simulink model "inverse_dynamics_2dof_PID"  (R2023b)
settings: Solver=VariableStepAuto  StartTime=0.0  StopTime=Tend_slk  RelTol=1e-3
values from neighbouring files (symbols this model uses):
  Kd11 = 0.01333    [main_inverse_2dof_PID.m]
  Kd22 = 0.01333    [main_inverse_2dof_PID.m]
  Ki11 = 7.259e-10    [main_inverse_2dof_PID.m]
  Ki22 = 7.259e-10    [main_inverse_2dof_PID.m]
  Kp11 = 6.221e-06    [main_inverse_2dof_PID.m]
  Kp22 = 6.221e-06    [main_inverse_2dof_PID.m]
  param = [Ixx;Iyy;Izz;l;k1;k2;k3;k4;b;m]    [main_inverse_2dof_PID.m]
  Ts_slk = 0.01    [main_inverse_2dof_PID.m]
  x0 = [0;0;0;0]    [main_inverse_2dof_PID.m]
undefined symbols (not defined in the file or in its folder): x_eq
libraries: slpidlib x2, cstblocks x1
settings Model: Creator=asus  LastModifiedBy=asus
settings OptimizationCC: ReuseModelBlockBuffer=off

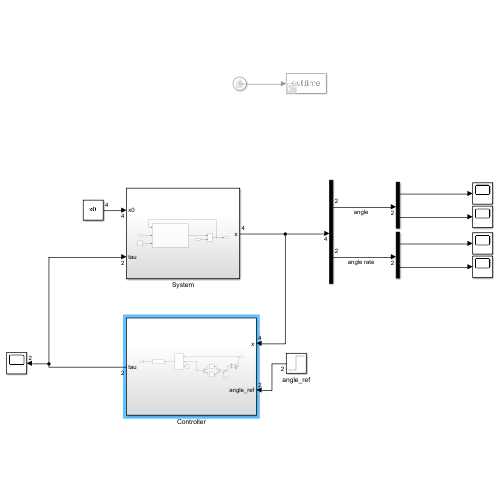
[thumbnail: Simulink's stored preview of the top-level diagram]
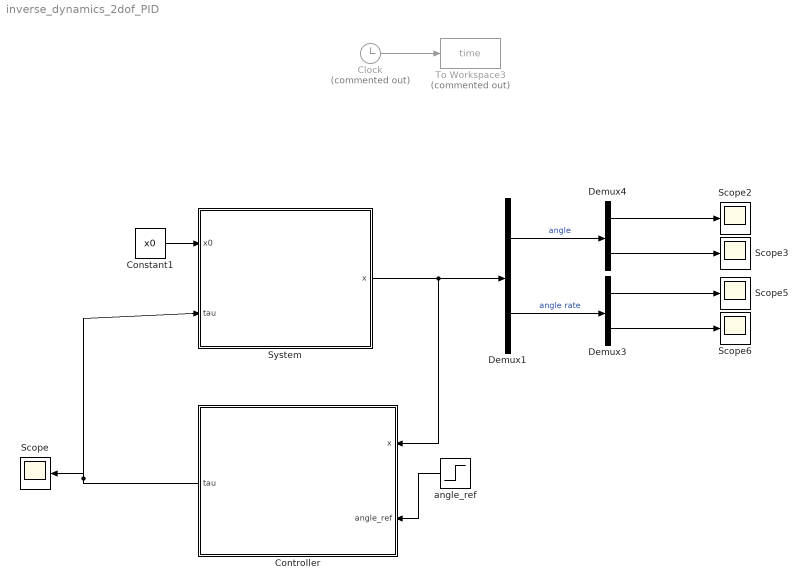
== system inverse_dynamics_2dof_PID ==
  Clock : Clock  Commented=on
  Constant1 : Constant  Value=x0
  Controller : Subsystem
  Demux1 : Demux  Outputs=2
  Demux3 : Demux  Outputs=2
  Demux4 : Demux  Outputs=2
  Scope{,2..3,5..6} (5 alike) : Scope
  System : Subsystem
  To Workspace3 : ToWorkspace  Commented=on  VariableName=time  SampleTime=Ts_slk
      settings: Save2DSignal=2-D array (concatenate along first dimension)
  angle_ref : Step  Time=0  After=[1;1]*30*pi/180  SampleTime=0
  wires:
  Clock/1 -> To Workspace3/1
  Demux4/1 -> Scope2/1
  Demux3/1 -> Scope5/1
  Demux4/2 -> Scope3/1
  Demux3/2 -> Scope6/1
  System/1(x) -> Controller/1(x), Demux1/1
  Demux1/2 -> Demux3/1  "angle rate"
  Demux1/1 -> Demux4/1  "angle"
  Controller/1(tau) -> Scope/1, System/2("tau ")
  angle_ref/1 -> Controller/2(angle_ref)
  Constant1/1 -> System/1(x0)

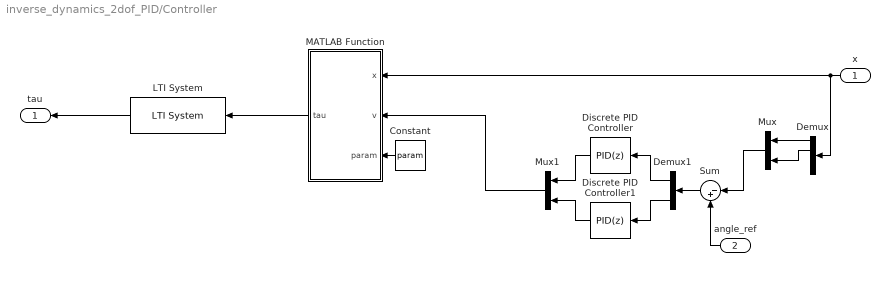
== system inverse_dynamics_2dof_PID/Controller ==
  x : Inport
  angle_ref : Inport  Port=2
  Constant : Constant  Value=param
  Demux : Demux
  Demux1 : Demux  Outputs=2
  Discrete PID Controller : slpidlib/PID Controller  Controller=PID  Form=Parallel  TimeDomain=Discrete-time  UseExternalTs=off  SampleTime=-1  IntegratorMethod=Forward Euler  FilterMethod=Forward Euler  ControllerParametersSource=internal  P=Kp11  I=Ki11  UseKiTs=off  D=Kd11  N=100  UseFilter=on  TunerSelectOption=Transfer Function Based (PID Tuner App)  InitialConditionSource=internal  InitialConditionForIntegrator=0  InitialConditionForFilter=0  DifferentiatorICPrevScaledInput=0  ExternalReset=none  TrackingMode=off  Kt=1  LimitOutput=off  SatLimitsSource=internal  UpperSaturationLimit=inf  LowerSaturationLimit=-inf  LinearizeAsGain=off  AntiWindupMode=none  Kb=1  LimitIntegrator=off  UpperIntegratorSaturationLimit=inf  LowerIntegratorSaturationLimit=-inf  POutMin=[]  POutMax=[]  IOutMin=[]  IOutMax=[]  DOutMin=[]  DOutMax=[]  NOutMin=[]  NOutMax=[]  SumOutMin=[]  SumOutMax=[]  SaturationOutMin=[]  SaturationOutMax=[]  PParamMin=[]  PParamMax=[]  IParamMin=[]  IParamMax=[]  DParamMin=[]  DParamMax=[]  NParamMin=[]  NParamMax=[]  KbParamMin=[]  KbParamMax=[]  KtParamMin=[]  KtParamMax=[]  KbOutMin=[]  KbOutMax=[]  KtOutMin=[]  KtOutMax=[]  IntegratorOutMin=[]  IntegratorOutMax=[]  FilterOutMin=[]  FilterOutMax=[]  SumI1OutMin=[]  SumI1OutMax=[]  SumI2OutMin=[]  SumI2OutMax=[]  SumI3OutMin=[]  SumI3OutMax=[]  SumI4OutMin=[]  SumI4OutMax=[]  SumDOutMin=[]  SumDOutMax=[]  DifferentiatorOutMin=[]  DifferentiatorOutMax=[]  FilterDiffOutCoefMin=[]  FilterDiffOutCoefMax=[]  ReciprocalOutMin=[]  ReciprocalOutMax=[]  SumDenOutMin=[]  SumDenOutMax=[]  SumNumOutMin=[]  SumNumOutMax=[]  DivideOutMin=[]  DivideOutMax=[]  UdiffTsProdOutMin=[]  UdiffTsProdOutMax=[]  NTsProdOutMin=[]  NTsProdOutMax=[]  UintegralTsProdOutMin=[]  UintegralTsProdOutMax=[]  UngainTsProdOutMin=[]  UngainTsProdOutMax=[]  ClampingZeroOutDataTypeStr=Inherit: Inherit via back propagation  ClampingZeroOutMin=[]  ClampingZeroOutMax=[]  FilterDenConstantOutDataTypeStr=Inherit: Inherit via back propagation  FilterDenConstantOutMin=[]  FilterDenConstantOutMax=[]  PCopyOutDataTypeStr=Inherit: Inherit via back propagation  PCopyOutMin=[]  PCopyOutMax=[]  NCopyOutDataTypeStr=Inherit: Inherit via back propagation  NCopyOutMin=[]  NCopyOutMax=[]  IntegratorContinuousStateAttributes=''  IntegratorStateMustResolveToSignalObject=off  IntegratorRTWStateStorageClass=Auto  FilterContinuousStateAttributes=''  FilterStateMustResolveToSignalObject=off  FilterRTWStateStorageClass=Auto  ParallelPVariant=InternalParameters  IdealPVariant=Disabled  IVariant=InternalParameters  DVariant=InternalParameters  IntegratorVariant=Discrete  SatVariant=Disabled  AWVariant=Passthrough  PCopyVariant=Disabled  TRVariant=Disabled  FdbkBlocksVariant=Forward  IdealPFdbkVariant=Disabled  SatFdbkVariant=Disabled  DerivativeFilterVariant=ForwardEulerFilter  NVariant=InternalParameters  NCopyVariant=Disabled  FilterICVariant=InternalICsFilter  IntegratorICVariant=InternalICs  ExternalResetVariant=Disabled  TRSumVariant=Passthrough  SumFdbkVariant=Disabled  SumVariant=Sum_PID  TsampFilterVariant=InternalTs  TsampNgainVariant=Passthrough  TsampIntegralVariant=Disabled_SignalSpec  ExternalSaturationOutDataTypeStr=Inherit: Same as second input
      settings: LibrarySourceBlock=simulink/Discrete/Discrete PID Controller
  Discrete PID Controller1 : slpidlib/PID Controller  Controller=PID  Form=Parallel  TimeDomain=Discrete-time  UseExternalTs=off  SampleTime=-1  IntegratorMethod=Forward Euler  FilterMethod=Forward Euler  ControllerParametersSource=internal  P=Kp22  I=Ki22  UseKiTs=off  D=Kd22  N=100  UseFilter=on  TunerSelectOption=Transfer Function Based (PID Tuner App)  InitialConditionSource=internal  InitialConditionForIntegrator=0  InitialConditionForFilter=0  DifferentiatorICPrevScaledInput=0  ExternalReset=none  TrackingMode=off  Kt=1  LimitOutput=off  SatLimitsSource=internal  UpperSaturationLimit=inf  LowerSaturationLimit=-inf  LinearizeAsGain=off  AntiWindupMode=none  Kb=1  LimitIntegrator=off  UpperIntegratorSaturationLimit=inf  LowerIntegratorSaturationLimit=-inf  POutMin=[]  POutMax=[]  IOutMin=[]  IOutMax=[]  DOutMin=[]  DOutMax=[]  NOutMin=[]  NOutMax=[]  SumOutMin=[]  SumOutMax=[]  SaturationOutMin=[]  SaturationOutMax=[]  PParamMin=[]  PParamMax=[]  IParamMin=[]  IParamMax=[]  DParamMin=[]  DParamMax=[]  NParamMin=[]  NParamMax=[]  KbParamMin=[]  KbParamMax=[]  KtParamMin=[]  KtParamMax=[]  KbOutMin=[]  KbOutMax=[]  KtOutMin=[]  KtOutMax=[]  IntegratorOutMin=[]  IntegratorOutMax=[]  FilterOutMin=[]  FilterOutMax=[]  SumI1OutMin=[]  SumI1OutMax=[]  SumI2OutMin=[]  SumI2OutMax=[]  SumI3OutMin=[]  SumI3OutMax=[]  SumI4OutMin=[]  SumI4OutMax=[]  SumDOutMin=[]  SumDOutMax=[]  DifferentiatorOutMin=[]  DifferentiatorOutMax=[]  FilterDiffOutCoefMin=[]  FilterDiffOutCoefMax=[]  ReciprocalOutMin=[]  ReciprocalOutMax=[]  SumDenOutMin=[]  SumDenOutMax=[]  SumNumOutMin=[]  SumNumOutMax=[]  DivideOutMin=[]  DivideOutMax=[]  UdiffTsProdOutMin=[]  UdiffTsProdOutMax=[]  NTsProdOutMin=[]  NTsProdOutMax=[]  UintegralTsProdOutMin=[]  UintegralTsProdOutMax=[]  UngainTsProdOutMin=[]  UngainTsProdOutMax=[]  ClampingZeroOutDataTypeStr=Inherit: Inherit via back propagation  ClampingZeroOutMin=[]  ClampingZeroOutMax=[]  FilterDenConstantOutDataTypeStr=Inherit: Inherit via back propagation  FilterDenConstantOutMin=[]  FilterDenConstantOutMax=[]  PCopyOutDataTypeStr=Inherit: Inherit via back propagation  PCopyOutMin=[]  PCopyOutMax=[]  NCopyOutDataTypeStr=Inherit: Inherit via back propagation  NCopyOutMin=[]  NCopyOutMax=[]  IntegratorContinuousStateAttributes=''  IntegratorStateMustResolveToSignalObject=off  IntegratorRTWStateStorageClass=Auto  FilterContinuousStateAttributes=''  FilterStateMustResolveToSignalObject=off  FilterRTWStateStorageClass=Auto  ParallelPVariant=InternalParameters  IdealPVariant=Disabled  IVariant=InternalParameters  DVariant=InternalParameters  IntegratorVariant=Discrete  SatVariant=Disabled  AWVariant=Passthrough  PCopyVariant=Disabled  TRVariant=Disabled  FdbkBlocksVariant=Forward  IdealPFdbkVariant=Disabled  SatFdbkVariant=Disabled  DerivativeFilterVariant=ForwardEulerFilter  NVariant=InternalParameters  NCopyVariant=Disabled  FilterICVariant=InternalICsFilter  IntegratorICVariant=InternalICs  ExternalResetVariant=Disabled  TRSumVariant=Passthrough  SumFdbkVariant=Disabled  SumVariant=Sum_PID  TsampFilterVariant=InternalTs  TsampNgainVariant=Passthrough  TsampIntegralVariant=Disabled_SignalSpec  ExternalSaturationOutDataTypeStr=Inherit: Same as second input
      settings: LibrarySourceBlock=simulink/Discrete/Discrete PID Controller
  LTI System : cstblocks/LTI System  sys=Decoupler_disc  IC=[]  PadeOrder=0
  MATLAB Function : MATLAB Function  TreatAsAtomicUnit=on
  Mux : Mux  Inputs=2
  Mux1 : Mux  Inputs=2
  Sum : Sum  Inputs=|-+
  tau : Outport
  wires:
  Constant/1 -> MATLAB Function/3(param)
  x/1 -> Demux/1, MATLAB Function/1(x)
  Sum/1 -> Demux1/1
  angle_ref/1 -> Sum/2
  Demux/1 -> Mux/1
  Mux/1 -> Sum/1
  Demux1/1 -> Discrete PID Controller/1
  Demux1/2 -> Discrete PID Controller1/1
  Discrete PID Controller/1 -> Mux1/1
  Discrete PID Controller1/1 -> Mux1/2
  Demux/2 -> Mux/2
  MATLAB Function/1(tau) -> LTI System/1
  LTI System/1 -> tau/1
  Mux1/1 -> MATLAB Function/2(v)

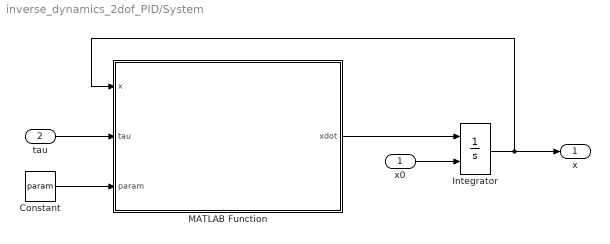
== system inverse_dynamics_2dof_PID/System ==
  x0 : Inport
  "tau " : Inport  Port=2
  Constant : Constant  Value=param
  Integrator : Integrator  InitialConditionSource=external  InitialCondition=x_eq
  MATLAB Function : MATLAB Function  TreatAsAtomicUnit=on
  x : Outport
  wires:
  Integrator/1 -> MATLAB Function/1(x), x/1
  MATLAB Function/1(xdot) -> Integrator/1
  "tau "/1 -> MATLAB Function/2(tau)
  Constant/1 -> MATLAB Function/3(param)
  x0/1 -> Integrator/2

== matlab function inverse_dynamics_2dof_PID/System/MATLAB Function ==
  data: x input; tau input; xdot output; param input
function xdot=quadcopter(x,tau,param)
% Inputs:
%           x       (model state)
%           tau     (torque)           
%           param   (model parameters)
%
% Outputs:  x_dot  (derivative of the state with respect to time)

% Parameters
g        =       9.81;           %  gravity acceleration (m/s^2)
Ixx      =       param(1,1);     %  moment of inertia 
Iyy      =       param(2,1);     %  moment of inertia
Izz      =       param(3,1);     %  moment of inertia 

% States
phi      =       x(1,1);     %  roll angle (rad)
theta    =       x(2,1);     %  pitch angle (rad)
phi_dot  =       x(3,1);     %  roll rate (rad/s)
theta_dot=       x(4,1);     %  pitch rate (rad/s)

cph         =       cos(phi);
cth         =       cos(theta);
sph         =       sin(phi);
sth         =       sin(theta);

% torques
tau_1    =       tau(1,1);   %  roll torque 
tau_2    =       tau(2,1);   %  pitch torque  

% Coriolis matrix
C11=  0;
C12= (Iyy)*(theta_dot*cph*sph);
C21= (Iyy)*(theta_dot*cph*sph);
C22= 0;

C  = [C11 C12;
      C21 C22];

% Inertia matrix
J11= Ixx;
J12= 0;
J21= 0;
J22= Iyy*cph^2;

J  = [J11 J12;
     J21 J22];

%% Model Equation 
invJ = [ J22/(J11*J22 - J12*J21), -J12/(J11*J22 - J12*J21);
        -J21/(J11*J22 - J12*J21),  J11/(J11*J22 - J12*J21)];

xdot        = zeros(4,1);
xdot(1:2,1) = x(3:4,1);
xdot(3:4,1) = invJ*(tau - C*x(3:4,1));

== matlab function inverse_dynamics_2dof_PID/Controller/MATLAB Function ==
  data: x input; v input; tau output; param input
function tau = fcn(x,v,param)
% Inputs:
%           x       (model state)
%           v       (new input to the feedback system)           
%           param   (model parameters)
%
% Outputs:  tau     (torque)

% Parameters
g        =       9.81;           %  gravity acceleration (m/s^2)
Ixx      =       param(1,1);     %  moment of inertia 
Iyy      =       param(2,1);     %  moment of inertia
Izz      =       param(3,1);     %  moment of inertia 

% States
phi      =       x(1,1);     %  roll angle (rad)
theta    =       x(2,1);     %  pitch angle (rad)
phi_dot  =       x(3,1);     %  roll rate (rad/s)
theta_dot=       x(4,1);     %  pitch rate (rad/s)

cph         =       cos(phi);
cth         =       cos(theta);
sph         =       sin(phi);
sth         =       sin(theta);

% Coriolis matrix
C11=  0;
C12= (Iyy)*(theta_dot*cph*sph);
C21= (Iyy)*(theta_dot*cph*sph);
C22= 0;

C  = [C11 C12;
      C21 C22];

% Inertia matrix
J11= Ixx;
J12= 0;
J21= 0;
J22= Iyy*cph^2;

J  = [J11 J12;
     J21 J22];

%% Control law
tau = zeros(2,1);
tau = J*v+C*x(3:4,1);
